simulink library "utility_service_lib"  (Simulink 8.1)
settings: Solver=ode45  StartTime=0.0  StopTime=10.0  RelTol=1e-3
values from neighbouring files (symbols this model uses):
  Ts = 100E-6    (= 0.0001)    [BANSHEE_init.m]
undefined symbols (not defined in the file or in its folder): Left, type, V
libraries: simulink x10, rtlab x10, RMS_lib x10, cables_lib x8, breaker_lib x4, transformer_lib x3, EasyGen3500_GensetSignalScaling_lib x2, PQFV_lib x2, Banshee_SEL751_Woodward_lib x1, SEL751_SignalScaling_lib x1, ssn_lib x1, TestSeq_slave_lib x1
settings Model: Creator=RE25624  LastModifiedBy=re25624

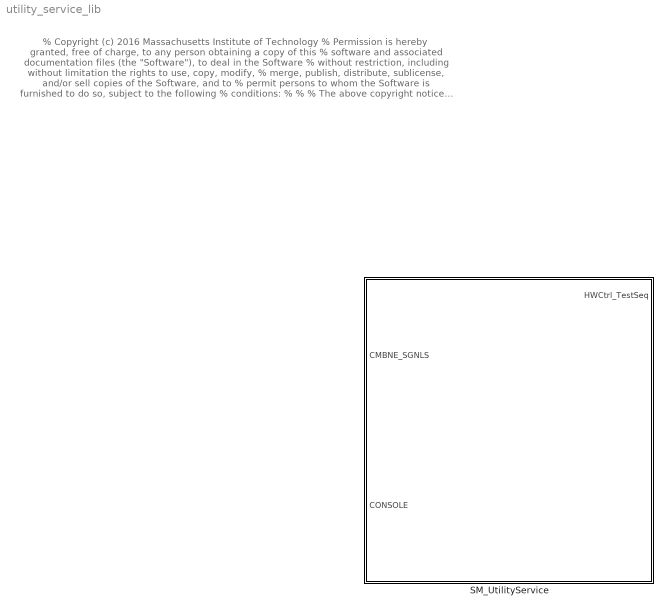
== system utility_service_lib ==
  note: % Copyright (c) 2016 Massachusetts Institute of Technology
      | % Permission is hereby granted, free of charge, to any person obtaining a copy of this
      | % software and associated documentation files (the "Software"), to deal in the Software
      | % without restriction, including without limitation the rights to use, copy, modify,
      | % merge, publish, distribute, sublicense, and/or sell copies of the Software, and to
      | % permit persons to whom the Software is furnished to do so, subject to the following
      | % conditions:
      | %
      | %
      | % The above copyright notice and this permission notice shall be included in
      | % all copies or substantial portions of the Software.
      | %
      | % THE SOFTWARE IS PROVIDED "AS IS", WITHOUT WARRANTY OF ANY KIND, EXPRESS OR IMPLIED,
      | % INCLUDING BUT NOT LIMITED TO THE WARRANTIES OF MERCHANTABILITY, FITNESS FOR A
      | % PARTICULAR PURPOSE AND NONINFRINGEMENT. IN NO EVENT SHALL THE AUTHORS OR COPYRIGHT
      | % HOLDERS BE LIABLE FOR ANY CLAIM, DAMAGES OR OTHER LIABILITY, WHETHER IN AN ACTION
      | % OF CONTRACT, TORT OR OTHERWISE, ARISING FROM, OUT OF OR IN CONNECTION WITH THE
      | % SOFTWARE OR THE USE OR OTHER DEALINGS IN THE SOFTWARE.
      | %
      | %
      | %%
  SM_UtilityService : Subsystem

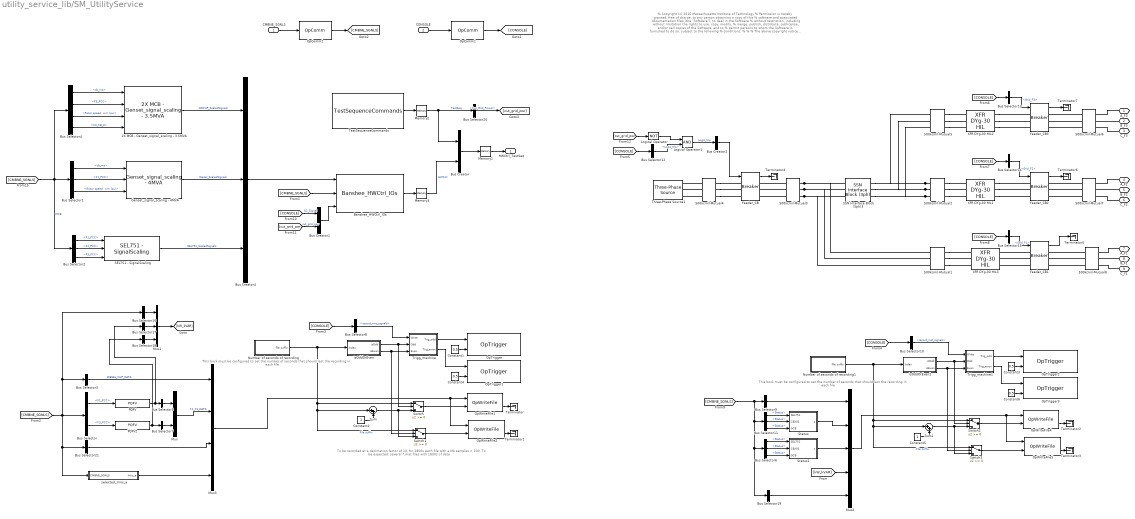
== system utility_service_lib/SM_UtilityService ==
  note: This bock must be configured to set the number of
      | seconds that should last the recording in each file
  note: To be recorded at a decimation factor of 10,   for 1800s each file with a Nb samples = 200.
      | To be expected: several *.mat files with 1800s of data
  note: This bock must be configured to set the number of
      | seconds that should last the recording in each file
  note: % Copyright (c) 2016 Massachusetts Institute of Technology
      | % Permission is hereby granted, free of charge, to any person obtaining a copy of this
      | % software and associated documentation files (the "Software"), to deal in the Software
      | % without restriction, including without limitation the rights to use, copy, modify,
      | % merge, publish, distribute, sublicense, and/or sell copies of the Software, and to
      | % permit persons to whom the Software is furnished to do so, subject to the following
      | % conditions:
      | %
      | %
      | % The above copyright notice and this permission notice shall be included in
      | % all copies or substantial portions of the Software.
      | %
      | % THE SOFTWARE IS PROVIDED "AS IS", WITHOUT WARRANTY OF ANY KIND, EXPRESS OR IMPLIED,
      | % INCLUDING BUT NOT LIMITED TO THE WARRANTIES OF MERCHANTABILITY, FITNESS FOR A
      | % PARTICULAR PURPOSE AND NONINFRINGEMENT. IN NO EVENT SHALL THE AUTHORS OR COPYRIGHT
      | % HOLDERS BE LIABLE FOR ANY CLAIM, DAMAGES OR OTHER LIABILITY, WHETHER IN AN ACTION
      | % OF CONTRACT, TORT OR OTHERWISE, ARISING FROM, OUT OF OR IN CONNECTION WITH THE
      | % SOFTWARE OR THE USE OR OTHER DEALINGS IN THE SOFTWARE.
      | %
      | %
      | %%
  CMBNE_SGNLS : Inport
  CONSOLE : Inport  Port=2
  2X MCB - Genset_signal_scaling - 3.5MVA : EasyGen3500_GensetSignalScaling_lib/2X MCB - Genset_signal_scaling - 3.5MVA  Vpk_mcb=11268  watt_mcb=3150000  Vpk_gcb=11268  watt_gcb=3150000  rated_rpm=1800  wm_noise_bias=0.02
  500kcmil-Mutual1 : cables_lib/500kcmil-Mutual  length=200  par_sets=1  ratio=3
  500kcmil-Mutual2 : cables_lib/500kcmil-Mutual  length=200  par_sets=1  ratio=3
  500kcmil-Mutual{3..4,6..8} (5 alike) : cables_lib/500kcmil-Mutual  length=50  par_sets=1  ratio=3
  500kcmil-Mutual5 : cables_lib/500kcmil-Mutual  length=200  par_sets=1  ratio=3
  Banshee_HWCtrl_IOs : Banshee_SEL751_Woodward_lib/Banshee_HWCtrl_IOs  SystemSampleTime=-1
  Bus Creator : BusCreator  Inputs=2
  Bus Creator1 : BusCreator  Inputs=2
  Bus Creator2 : BusCreator  Inputs=1
  Bus Creator4 : BusCreator  Inputs=3
  Bus Selector : BusSelector  OutputSignals=F1_MS_IN.CB_DATA.F1_PCC,F3_MS_IN.CB_DATA.F3_PCC
  Bus Selector1 : BusSelector  OutputSignals="F1_MS_IN.DIESEL_DATA.DIESEL_GCB.cb_ms,F1_MS_IN.CB_DATA.F1_PCC,F1_MS_IN.DIESEL_DATA.Gen2_meas.w.w.Rotor speed  wm (pu)"
  Bus Selector10 : BusSelector  OutputSignals=DataLogging.record_inst_signals
  Bus Selector11 : BusSelector  OutputSignals=F1_MS_IN.CB_DATA.F1_PCC.Status,F1_MS_IN.CB_DATA.F1_CB_3.Status,F1_MS_IN.DIESEL_DATA.DIESEL_GCB.cb_ms.Status
  Bus Selector12 : BusSelector  OutputSignals=GridStatusCtrl.Substation.Logic_trip
  Bus Selector13 : BusSelector  OutputSignals=GridStatusCtrl.Grid_F3
  Bus Selector14 : BusSelector  OutputSignals=GridStatusCtrl.Grid_F2
  Bus Selector15 : BusSelector  OutputSignals=GridStatusCtrl.Grid_F1
  Bus Selector16 : BusSelector  OutputSignals=F1_MS_IN.DIESEL_DATA.DIESEL_GCB.kw,F1_MS_IN.DIESEL_DATA.DIESEL_GCB.kvar,F3_MS_IN.NG_CHP_DATA.NG_CHP_GCB.kw,F3_MS_IN.NG_CHP_DATA.NG_CHP_GCB.kvar  OutputAsBus=on
  Bus Selector17 : BusSelector  OutputSignals=kw,kvar  OutputAsBus=on
  Bus Selector18 : BusSelector  OutputSignals=kw,kvar  OutputAsBus=on
  Bus Selector19 : BusSelector  OutputSignals=F1_MS_IN.DIESEL_DATA.DIESEL_GCB.cb_ms.Iabc,F3_MS_IN.NG_CHP_DATA.NG_CHP_GCB.cb_ms.Iabc,F1_MS_IN.DIESEL_DATA.Gen2_meas.Vf.vf,F3_MS_IN.NG_CHP_DATA.Gen1_meas.Vf.vf  OutputAsBus=on
  Bus Selector2 : BusSelector  OutputSignals=F1_MS_IN.CB_DATA.F1_PCC,F2_MS_IN.CB_DATA.F2_PCC,F3_MS_IN.CB_DATA.F3_PCC
  Bus Selector20 : BusSelector  OutputSignals=Cut_Grid_Power
  Bus Selector21 : BusSelector  OutputSignals=F1_RELAY_OUT.F1_CB_1.m.status,F1_RELAY_OUT.F1_CB_2.m.status,F1_RELAY_OUT.F1_CB_3.m.status,F1_RELAY_OUT.F1_CB_4.m.status,F1_RELAY_OUT.F1_CB_5.m.status,F1_RELAY_OUT.F1_CB_6.m.status,F1_RELAY_OUT.F1_CB_7.m.status,F1_RELAY_OUT.F1_CB_8.m.status,F1_RELAY_OUT.F1_CB_9.m.status,F1_RELAY_OUT.F1_CB_10.m.status,F1_RELAY_OUT.F1_CB_11.m.status,F1_RELAY_OUT.F1_CB_12.m.status,F1_RELAY_OUT.F1_CB_13.m.status,F1_RELAY_OUT.F1_CB_14.m.status,F2_RELAY_OUT.F2_CB_1.m.status,F2_RELAY_OUT.F2_CB_2.m.status,F2_RELAY_OUT.F2_CB_3.m.status,F2_RELAY_OUT.F2_CB_4.m.status,F2_RELAY_OUT.F2_CB_5.m.status,F2_RELAY_OUT.F2_CB_6.m.status,F2_RELAY_OUT.F2_CB_7.m.status,F2_RELAY_OUT.F2_CB_8.m.status,F2_RELAY_OUT.F2_CB_9.m.status,F2_RELAY_OUT.F2_CB_10.m.status,F2_RELAY_OUT.F2_CB_11.m.status,F2_RELAY_OUT.F2_CB_12.m.status,F2_RELAY_OUT.F2_CB_13.m.status,F2_RELAY_OUT.F2_CB_14.m.status,F2_RELAY_OUT.F2_CB_15.m.status,F2_RELAY_OUT.F2_CB_16.m.status,F2_RELAY_OUT.F2_CB_17.m.status,F2_RELAY_OUT.F2_CB_18.m.status,F2_RELAY_OUT.F2_CB_19.m.status,F3_RELAY_OUT.F3_CB_1.m.status,F3_RELAY_OUT.F3_CB_2.m.status,F3_RELAY_OUT.F3_CB_3.m.status,F3_RELAY_OUT.F3_CB_4.m.status,F3_RELAY_OUT.F3_CB_5.m.status,F3_RELAY_OUT.F3_CB_6.m.status,F3_RELAY_OUT.F3_CB_7.m.status,F3_RELAY_OUT.F3_CB_8.m.status,F3_RELAY_OUT.F3_CB_9.m.status  OutputAsBus=on
  Bus Selector3 : BusSelector  OutputSignals=F1_MS_IN.DIESEL_DATA.DIESEL_GCB.VRMSLL,F1_MS_IN.DIESEL_DATA.DIESEL_GCB.Freq,F1_MS_IN.DIESEL_DATA.DIESEL_GCB.kw,F1_MS_IN.DIESEL_DATA.DIESEL_GCB.kvar,F3_MS_IN.NG_CHP_DATA.NG_CHP_GCB.VRMSLL,F3_MS_IN.NG_CHP_DATA.NG_CHP_GCB.Freq,F3_MS_IN.NG_CHP_DATA.NG_CHP_GCB.kw,F3_MS_IN.NG_CHP_DATA.NG_CHP_GCB.kvar  OutputAsBus=on
  Bus Selector4 : BusSelector  OutputSignals="F3_MS_IN.NG_CHP_DATA.NG_CHP_GCB.cb_ms,F3_MS_IN.CB_DATA.F3_PCC,F3_MS_IN.NG_CHP_DATA.Gen1_meas.w.w.Rotor speed  wm (pu),F3_MS_IN.CB_DATA.F3_CB_3"
  Bus Selector5 : BusSelector  OutputSignals=VRMSLL,Freq,kw,kvar  OutputAsBus=on
  Bus Selector6 : BusSelector  OutputSignals=F3_MS_IN.CB_DATA.F3_PCC.Status,F3_MS_IN.CB_DATA.F3_CB_3.Status,F3_MS_IN.NG_CHP_DATA.NG_CHP_GCB.cb_ms.Status
  Bus Selector7 : BusSelector  OutputSignals=VRMSLL,Freq,kw,kvar  OutputAsBus=on
  Bus Selector8 : BusSelector  OutputSignals=DataLogging.record_rms_signals
  Bus Selector9 : BusSelector  OutputSignals=F1_MS_IN.CB_DATA.F1_PCC.Vabc_bus,F3_MS_IN.CB_DATA.F3_PCC.Vabc_bus,F1_MS_IN.DIESEL_DATA.DIESEL_GCB.cb_ms.Vabc_bus,F3_MS_IN.NG_CHP_DATA.NG_CHP_GCB.cb_ms.Vabc_bus  OutputAsBus=on
  Constant{1,3..4,6} (4 alike) : Constant  Value=0.5
  Constant2 : Constant
  Constant5 : Constant
  Feeder_CB{,1..3} (4 alike) : breaker_lib/Breaker  Ts=Ts  mech_delay=cb_mech_delay
  Genset_signal_scaling - 4MVA : EasyGen3500_GensetSignalScaling_lib/Genset_signal_scaling - 4MVA  Vpk_mcb=11268  watt_mcb=3600000  Vpk_gcb=11268  watt_gcb=3600000  rated_rpm=1800  wm_noise_bias=0.02
  Logical Operator : Logic  Operator=NOT  AllPortsSameDT=off  OutDataTypeStr=boolean
  Logical Operator1 : Logic  AllPortsSameDT=off  OutDataTypeStr=boolean
  Memory1 : Memory
  Memory2 : Memory
  Memory3 : Memory
  Mux : Mux  Inputs=2
  Mux1 : Mux  Inputs=3
  Mux2 : Mux  Inputs=5
  Mux3 : Mux
  Number of seconds of recording : Subsystem  mask{time_s=1800}
      mask prompts: time_s "Time in seconds"
      mask help: Set the number of seconds that should last the recording in each file.
  Number of seconds of recording1 : Subsystem  mask{time_s=300}
      mask prompts: time_s "Time in seconds"
      mask help: Set the number of seconds that should last the recording in each file.
  OpComm1 : rtlab/OpComm  nbport=1  groupe_acq=1  subsys_rate=0  st=0  Synchronization=on  Interpolation=on  Threshold=1.0  Missed_Data=off  Sim_Time=off  Samples=off  dynSigOut=off  from_console=1  warning_done=off  writeOpCommFile=off  Offset=off
  OpComm2 : rtlab/OpComm  nbport=1  groupe_acq=1  subsys_rate=0  st=0  Synchronization=on  Interpolation=on  Threshold=1.0  Missed_Data=off  Sim_Time=off  Samples=off  dynSigOut=off  from_console=0  warning_done=off  writeOpCommFile=off  Offset=off
  OpTrigger : rtlab/DataLogging/OpTrigger  Trig_Type=TRIGGER SIGNAL >= TRIGGER LEVEL  Trig_Offset=0  Acq_Group=28
  OpTrigger1 : rtlab/DataLogging/OpTrigger  Trig_Type=TRIGGER SIGNAL >= TRIGGER LEVEL  Trig_Offset=0  Acq_Group=29
  OpTrigger2 : rtlab/DataLogging/OpTrigger  Trig_Type=TRIGGER SIGNAL >= TRIGGER LEVEL  Trig_Offset=0  Acq_Group=26
  OpTrigger3 : rtlab/DataLogging/OpTrigger  Trig_Type=TRIGGER SIGNAL >= TRIGGER LEVEL  Trig_Offset=0  Acq_Group=27
  OpWriteFile1 : rtlab/DataLogging/OpWriteFile  Static_File=off  varname=recVar  Filename=A_FILE_RECORDED_o.mat  rtpath='./'  nrtpath='.\'  Acq_Group=28  file_size=150000000  write_offline=off  Sim_Mode=off  Nb_Samples=1000  Buffer_size=0
      settings: Decimation=20
  OpWriteFile2 : rtlab/DataLogging/OpWriteFile  Static_File=off  varname=recVar  Filename=A_FILE_RECORDED_e.mat  rtpath='./'  nrtpath='.\'  Acq_Group=29  file_size=150000000  write_offline=off  Sim_Mode=off  Nb_Samples=1000  Buffer_size=0
      settings: Decimation=20
  OpWriteFile4 : rtlab/DataLogging/OpWriteFile  Static_File=off  varname=recVar  Filename=A_INST_RECORDED_o.mat  rtpath='./'  nrtpath='.\'  Acq_Group=26  file_size=150000000  write_offline=off  Sim_Mode=off  Nb_Samples=1000  Buffer_size=0
      settings: Decimation=4
  OpWriteFile5 : rtlab/DataLogging/OpWriteFile  Static_File=off  varname=recVar  Filename=A_INST_RECORDED_e.mat  rtpath='./'  nrtpath='.\'  Acq_Group=27  file_size=150000000  write_offline=off  Sim_Mode=off  Nb_Samples=1000  Buffer_size=0
      settings: Decimation=4
  PQFV : PQFV_lib/PQFV  VRMSLL=13800
  PQFV2 : PQFV_lib/PQFV  VRMSLL=13800
  SEL751 - SignalScaling : SEL751_SignalScaling_lib/SEL751 - SignalScaling  ct_ratio=1/1250  pt_ratio=1/1800
  SSN Interface Block (3ph)3 : ssn_lib/SSN Interface Block (3ph)  nb_phase=3  nb_port=2  p1_type=V-type(Left)  p2_type=V-type (Right)  p3_type=V-type(Left)  p4_type=V-type(Left)  p5_type=V-type(Left)  p6_type=V-type(Left)  p7_type=V-type(Left)  p8_type=V-type(Left)  p9_type=V-type(Left)  p10_type=V-type(Left)  p11_type=V-type(Left)  p12_type=V-type(Left)  p13_type=V-type(Left)  p14_type=V-type(Left)  p15_type=V-type(Left)  p16_type=V-type(Left)  I_port_shunt_resistance=1e9
  Status : Subsystem
  Status1 : Subsystem
  Sum : Sum  Inputs=|++
  Sum1 : Sum  Inputs=|++
  Switch{,1..3} (4 alike) : Switch
  Terminator{,1..7} (8 alike) : Terminator
  TestSequenceCommands : TestSeq_slave_lib/TestSequenceCommands
  Three-Phase Source1 : powerlib/Electrical Sources/Three-Phase Source  Voltage=115000  PhaseAngle=0  Frequency=60  InternalConnection=Yg  SpecifyImpedance=on  Resistance=0.8929  Inductance=16.58e-3  ShortCircuitLevel=2000e6  BaseVoltage=115000  XRratio=100  BusType=swing  Pref=0  Qref=0  Qmin=-inf  Qmax=inf
  Trigg_machine : Subsystem
  Trigg_machine1 : Subsystem
  XFR DYg-30 HIL1 : transformer_lib/XFR DYg-30 HIL  Rating=50000  Vp=115000  Vs=13800  Z=6  XR=30
  XFR DYg-30 HIL2 : transformer_lib/XFR DYg-30 HIL  Rating=50000  Vp=115000  Vs=13800  Z=6  XR=30
  XFR DYg-30 HIL3 : transformer_lib/XFR DYg-30 HIL  Rating=50000  Vp=115000  Vs=13800  Z=6  XR=30
  isOddOrEven : Subsystem
  isOddOrEven1 : Subsystem
  selected_Irms_a : Subsystem
  A_F3 : PMIOPort  Port=1  Side=Right
  B_F3 : PMIOPort  Port=2  Side=Right
  C_F3 : PMIOPort  Port=3  Side=Right
  A_F2 : PMIOPort  Port=4  Side=Right
  B_F2 : PMIOPort  Port=5  Side=Right
  C_F2 : PMIOPort  Port=6  Side=Right
  A_F1 : PMIOPort  Port=7  Side=Right
  B_F1 : PMIOPort  Port=8  Side=Right
  C_F1 : PMIOPort  Port=9  Side=Right
  HWCtrl_TestSeq : Outport
  wires:
  Bus Creator2/1 -> Feeder_CB/1
  Logical Operator1/1 -> Bus Creator2/1  "Logic_trip"
  Logical Operator/1 -> Logical Operator1/1
  [cut_grid_pwr] -> Logical Operator/1
  [cut_grid_pwr] -> Bus Creator1/2  "cut_grid_pwr"
  Bus Selector20/1 -> [cut_grid_pwr]  "<Cut_Grid_Power>"
  Bus Creator1/1 -> Banshee_HWCtrl_IOs/3
  selected_Irms_a/1(Irms_a) -> Mux3/4
  Bus Creator/1 -> Memory1/1
  Memory2/1 -> Bus Selector20/1, Bus Creator/1  "TestSeq"
  Memory3/1 -> Bus Creator/2  "HWCtrl"
  TestSequenceCommands/1 -> Memory2/1
  Banshee_HWCtrl_IOs/1 -> Memory3/1
  Memory1/1 -> HWCtrl_TestSeq/1
  Bus Selector21/1 -> Mux3/3
  Bus Selector19/1 -> Mux2/5
  [kW_kVAR] -> Mux2/4
  Mux1/1 -> [kW_kVAR]
  Bus Selector18/1 -> Mux1/3
  Bus Selector17/1 -> Mux1/2
  Bus Selector16/1 -> Mux1/1
  PQFV2/1 -> Bus Selector7/1, Bus Selector18/1
  PQFV/1 -> Bus Selector5/1, Bus Selector17/1
  Status1/1(o) -> Mux2/3
  Status/1(o) -> Mux2/2
  Bus Selector6/3 -> Status1/3(GCB)  "<Status>"
  Bus Selector6/2 -> Status1/2(CBX03)  "<Status>"
  Bus Selector6/1 -> Status1/1(SEL751)  "<Status>"
  Bus Selector11/3 -> Status/3(GCB)  "<Status>"
  Bus Selector11/2 -> Status/2(CBX03)  "<Status>"
  Bus Selector11/1 -> Status/1(SEL751)  "<Status>"
  [CONSOLE] -> Bus Creator1/1  "SC_Signal"
  Bus Selector9/1 -> Mux2/1
  [CMBNE_SGNLS] -> Bus Selector9/1, Bus Selector11/1, Bus Selector6/1, Bus Selector19/1
  Bus Selector15/1 -> Feeder_CB1/1  "<Grid_F1>"
  Bus Selector14/1 -> Feeder_CB2/1  "<Grid_F2>"
  Bus Selector13/1 -> Feeder_CB3/1  "<Grid_F3>"
  Bus Selector12/1 -> Logical Operator1/2  "<Logic_trip>"
  Feeder_CB3/1 -> Terminator7/1
  Feeder_CB2/1 -> Terminator6/1
  Feeder_CB1/1 -> Terminator5/1
  [CONSOLE] -> Bus Selector15/1
  [CONSOLE] -> Bus Selector14/1
  [CONSOLE] -> Bus Selector13/1
  [CONSOLE] -> Bus Selector12/1
  Feeder_CB/1 -> Terminator4/1
  [CMBNE_SGNLS] -> Bus Selector/1, Bus Selector21/1, selected_Irms_a/1(CMBNE_SGNLS), Bus Selector3/1, Bus Selector16/1
  [CONSOLE] -> Bus Selector10/1
  OpWriteFile5/2 -> Terminator3/1
  OpWriteFile4/2 -> Terminator2/1
  Bus Selector10/1 -> Trigg_machine1/1(Write)  "<record_inst_signals>"
  Number of seconds of recording1/1(file suffix) -> isOddOrEven1/1(Index), Sum1/1, Switch3/1, Switch2/1  "File suffix"
  Sum1/1 -> Switch2/3, Switch3/3
  Constant5/1 -> Sum1/2
  Switch3/1 -> OpWriteFile5/2
  Switch2/1 -> OpWriteFile4/2
  isOddOrEven1/2(isEven) -> Switch3/2, Trigg_machine1/3(Even)
  isOddOrEven1/1(isOdd) -> Switch2/2, Trigg_machine1/2(Odd)
  Constant6/1 -> OpTrigger3/2
  Constant3/1 -> OpTrigger2/2
  Trigg_machine1/2(Trig_even) -> OpTrigger3/1
  Trigg_machine1/1(Trig_odd) -> OpTrigger2/1
  Mux2/1 -> OpWriteFile4/1, OpWriteFile5/1
  [CONSOLE] -> Bus Selector8/1
  OpComm1/1 -> [CONSOLE]
  CONSOLE/1 -> OpComm1/1
  Mux/1 -> Mux3/2  "F1_F3_DATA"
  Bus Selector3/1 -> Mux3/1  "DIESEL_CHP_DATA"
  Bus Selector5/1 -> Mux/1
  Bus Selector7/1 -> Mux/2
  Bus Selector/2 -> PQFV2/1  "<F3_PCC>"
  Bus Selector/1 -> PQFV/1  "<F1_PCC>"
  OpWriteFile2/2 -> Terminator1/1
  OpWriteFile1/2 -> Terminator/1
  Bus Selector8/1 -> Trigg_machine/1(Write)  "<record_rms_signals>"
  Number of seconds of recording/1(file suffix) -> isOddOrEven/1(Index), Sum/1, Switch1/1, Switch/1  "File suffix"
  Sum/1 -> Switch/3, Switch1/3
  Constant2/1 -> Sum/2
  Switch1/1 -> OpWriteFile2/2
  Switch/1 -> OpWriteFile1/2
  isOddOrEven/2(isEven) -> Switch1/2, Trigg_machine/3(Even)
  isOddOrEven/1(isOdd) -> Switch/2, Trigg_machine/2(Odd)
  Constant4/1 -> OpTrigger1/2
  Constant1/1 -> OpTrigger/2
  Trigg_machine/2(Trig_even) -> OpTrigger1/1
  Trigg_machine/1(Trig_odd) -> OpTrigger/1
  Mux3/1 -> OpWriteFile1/1, OpWriteFile2/1
  [CMBNE_SGNLS] -> Banshee_HWCtrl_IOs/2
  Bus Selector4/4 -> 2X MCB - Genset_signal_scaling - 3.5MVA/4  "<F3_CB_3>"
  Bus Selector2/3 -> SEL751 - SignalScaling/3  "<F3_PCC>"
  Bus Selector2/1 -> SEL751 - SignalScaling/1  "<F1_PCC>"
  Bus Selector2/2 -> SEL751 - SignalScaling/2  "<F2_PCC>"
  SEL751 - SignalScaling/1 -> Bus Creator4/3  "SEL751_ScaledSignals"
  OpComm2/1 -> [CMBNE_SGNLS]
  CMBNE_SGNLS/1 -> OpComm2/1
  Bus Selector1/1 -> Genset_signal_scaling - 4MVA/1  "<cb_ms>"
  Bus Selector1/2 -> Genset_signal_scaling - 4MVA/2  "<F1_PCC>"
  Bus Selector1/3 -> Genset_signal_scaling - 4MVA/3  "<Rotor speed  wm (pu)>"
  Bus Creator4/1 -> Banshee_HWCtrl_IOs/1
  Bus Selector4/1 -> 2X MCB - Genset_signal_scaling - 3.5MVA/1  "<cb_ms>"
  Bus Selector4/2 -> 2X MCB - Genset_signal_scaling - 3.5MVA/2  "<F3_PCC>"
  Bus Selector4/3 -> 2X MCB - Genset_signal_scaling - 3.5MVA/3  "<Rotor speed  wm (pu)>"
  [CMBNE_SGNLS] -> Bus Selector1/1, Bus Selector2/1, Bus Selector4/1  "MCB"
  Genset_signal_scaling - 4MVA/1 -> Bus Creator4/2  "Diesel_ScaledSignals"
  2X MCB - Genset_signal_scaling - 3.5MVA/1 -> Bus Creator4/1  "NGCHP_ScaledSignals"
  connections:
  C_F3/RConn1 -- 500kcmil-Mutual6/RConn3
  A_F3/RConn1 -- 500kcmil-Mutual6/RConn1
  B_F3/RConn1 -- 500kcmil-Mutual6/RConn2
  C_F2/RConn1 -- 500kcmil-Mutual7/RConn3
  A_F2/RConn1 -- 500kcmil-Mutual7/RConn1
  B_F2/RConn1 -- 500kcmil-Mutual7/RConn2
  A_F1/RConn1 -- 500kcmil-Mutual8/RConn1
  C_F1/RConn1 -- 500kcmil-Mutual8/RConn3
  B_F1/RConn1 -- 500kcmil-Mutual8/RConn2
  500kcmil-Mutual8/LConn3 -- Feeder_CB1/RConn3
  500kcmil-Mutual8/LConn2 -- Feeder_CB1/RConn2
  500kcmil-Mutual8/LConn1 -- Feeder_CB1/RConn1
  500kcmil-Mutual7/LConn1 -- Feeder_CB2/RConn1
  500kcmil-Mutual7/LConn3 -- Feeder_CB2/RConn3
  500kcmil-Mutual7/LConn2 -- Feeder_CB2/RConn2
  500kcmil-Mutual6/LConn1 -- Feeder_CB3/RConn1
  500kcmil-Mutual6/LConn3 -- Feeder_CB3/RConn3
  500kcmil-Mutual6/LConn2 -- Feeder_CB3/RConn2
  Feeder_CB1/LConn1 -- XFR DYg-30 HIL3/RConn1
  Feeder_CB1/LConn2 -- XFR DYg-30 HIL3/RConn2
  Feeder_CB1/LConn3 -- XFR DYg-30 HIL3/RConn3
  XFR DYg-30 HIL1/RConn1 -- Feeder_CB2/LConn1
  XFR DYg-30 HIL1/RConn2 -- Feeder_CB2/LConn2
  XFR DYg-30 HIL1/RConn3 -- Feeder_CB2/LConn3
  XFR DYg-30 HIL2/RConn3 -- Feeder_CB3/LConn3
  XFR DYg-30 HIL2/RConn2 -- Feeder_CB3/LConn2
  XFR DYg-30 HIL2/RConn1 -- Feeder_CB3/LConn1
  500kcmil-Mutual2/LConn3 -- 500kcmil-Mutual5/LConn3 -- SSN Interface Block (3ph)3/RConn3
  500kcmil-Mutual2/LConn2 -- 500kcmil-Mutual5/LConn2 -- SSN Interface Block (3ph)3/RConn2
  500kcmil-Mutual2/LConn1 -- 500kcmil-Mutual5/LConn1 -- SSN Interface Block (3ph)3/RConn1
  500kcmil-Mutual1/RConn1 -- XFR DYg-30 HIL3/LConn1
  500kcmil-Mutual1/RConn2 -- XFR DYg-30 HIL3/LConn2
  500kcmil-Mutual1/RConn3 -- XFR DYg-30 HIL3/LConn3
  500kcmil-Mutual5/RConn3 -- XFR DYg-30 HIL2/LConn3
  500kcmil-Mutual5/RConn1 -- XFR DYg-30 HIL2/LConn1
  500kcmil-Mutual5/RConn2 -- XFR DYg-30 HIL2/LConn2
  500kcmil-Mutual2/RConn3 -- XFR DYg-30 HIL1/LConn3
  500kcmil-Mutual2/RConn1 -- XFR DYg-30 HIL1/LConn1
  500kcmil-Mutual2/RConn2 -- XFR DYg-30 HIL1/LConn2
  500kcmil-Mutual4/LConn2 -- Three-Phase Source1/RConn2
  500kcmil-Mutual4/LConn1 -- Three-Phase Source1/RConn1
  500kcmil-Mutual4/LConn3 -- Three-Phase Source1/RConn3
  500kcmil-Mutual4/RConn1 -- Feeder_CB/LConn1
  500kcmil-Mutual4/RConn2 -- Feeder_CB/LConn2
  500kcmil-Mutual4/RConn3 -- Feeder_CB/LConn3
  500kcmil-Mutual3/RConn3 -- 500kcmil-Mutual1/LConn3 -- SSN Interface Block (3ph)3/LConn3
  500kcmil-Mutual3/RConn1 -- 500kcmil-Mutual1/LConn1 -- SSN Interface Block (3ph)3/LConn1
  500kcmil-Mutual3/RConn2 -- 500kcmil-Mutual1/LConn2 -- SSN Interface Block (3ph)3/LConn2
  500kcmil-Mutual3/LConn2 -- Feeder_CB/RConn2
  500kcmil-Mutual3/LConn1 -- Feeder_CB/RConn1
  500kcmil-Mutual3/LConn3 -- Feeder_CB/RConn3

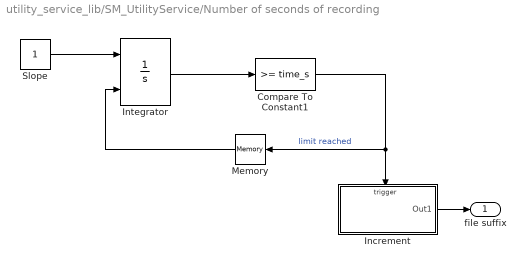
== system utility_service_lib/SM_UtilityService/Number of seconds of recording ==
  Compare To Constant1 : simulink/Logic and Bit Operations/Compare To Constant  relop=>=  const=time_s  OutDataTypeStr=boolean
  Increment : Subsystem
  Integrator : Integrator  ExternalReset=rising
  Memory : Memory
  Slope : Constant
  file suffix : Outport
  wires:
  Slope/1 -> Integrator/1
  Integrator/1 -> Compare To Constant1/1
  Compare To Constant1/1 -> Memory/1, Increment/Trigger  "limit reached"
  Memory/1 -> Integrator/2
  Increment/1(Out1) -> file suffix/1

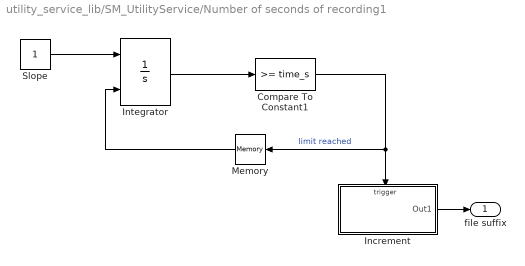
== system utility_service_lib/SM_UtilityService/Number of seconds of recording1 ==
  Compare To Constant1 : simulink/Logic and Bit Operations/Compare To Constant  relop=>=  const=time_s  OutDataTypeStr=boolean
  Increment : Subsystem
  Integrator : Integrator  ExternalReset=rising
  Memory : Memory
  Slope : Constant
  file suffix : Outport
  wires:
  Slope/1 -> Integrator/1
  Integrator/1 -> Compare To Constant1/1
  Compare To Constant1/1 -> Memory/1, Increment/Trigger  "limit reached"
  Memory/1 -> Integrator/2
  Increment/1(Out1) -> file suffix/1

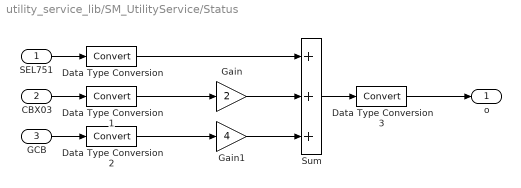
== system utility_service_lib/SM_UtilityService/Status ==
  SEL751 : Inport
  CBX03 : Inport  Port=2
  GCB : Inport  Port=3
  Data Type Conversion{,1..3} (4 alike) : DataTypeConversion
  Gain : Gain  Gain=2
  Gain1 : Gain  Gain=4
  Sum : Sum  Inputs=+++
  o : Outport
  wires:
  Data Type Conversion3/1 -> o/1
  Data Type Conversion2/1 -> Gain1/1
  Data Type Conversion1/1 -> Gain/1
  Data Type Conversion/1 -> Sum/1
  Sum/1 -> Data Type Conversion3/1
  Gain1/1 -> Sum/3
  Gain/1 -> Sum/2
  SEL751/1 -> Data Type Conversion/1
  CBX03/1 -> Data Type Conversion1/1
  GCB/1 -> Data Type Conversion2/1

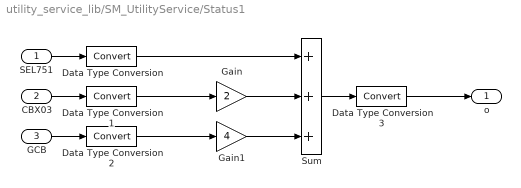
== system utility_service_lib/SM_UtilityService/Status1 ==
  SEL751 : Inport
  CBX03 : Inport  Port=2
  GCB : Inport  Port=3
  Data Type Conversion{,1..3} (4 alike) : DataTypeConversion
  Gain : Gain  Gain=2
  Gain1 : Gain  Gain=4
  Sum : Sum  Inputs=+++
  o : Outport
  wires:
  Data Type Conversion3/1 -> o/1
  Data Type Conversion2/1 -> Gain1/1
  Data Type Conversion1/1 -> Gain/1
  Data Type Conversion/1 -> Sum/1
  Sum/1 -> Data Type Conversion3/1
  Gain1/1 -> Sum/3
  Gain/1 -> Sum/2
  SEL751/1 -> Data Type Conversion/1
  CBX03/1 -> Data Type Conversion1/1
  GCB/1 -> Data Type Conversion2/1

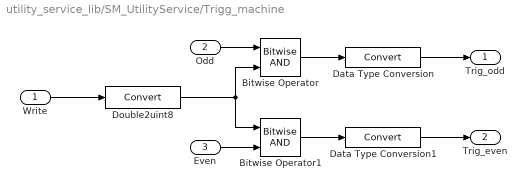
== system utility_service_lib/SM_UtilityService/Trigg_machine ==
  Write : Inport
  Odd : Inport  Port=2
  Even : Inport  Port=3
  Bitwise Operator : simulink/Logic and Bit Operations/Bitwise Operator  logicop=AND  UseBitMask=off  NumInputPorts=2  BitMask=bin2dec('11011001')  BitMaskRealWorld=Stored Integer
  Bitwise Operator1 : simulink/Logic and Bit Operations/Bitwise Operator  logicop=AND  UseBitMask=off  NumInputPorts=2  BitMask=bin2dec('11011001')  BitMaskRealWorld=Stored Integer
  Data Type Conversion : DataTypeConversion
  Data Type Conversion1 : DataTypeConversion
  Double2uint8 : DataTypeConversion
  Trig_odd : Outport
  Trig_even : Outport  Port=2
  wires:
  Double2uint8/1 -> Bitwise Operator1/1, Bitwise Operator/2
  Write/1 -> Double2uint8/1
  Odd/1 -> Bitwise Operator/1
  Data Type Conversion1/1 -> Trig_even/1
  Data Type Conversion/1 -> Trig_odd/1
  Even/1 -> Bitwise Operator1/2
  Bitwise Operator1/1 -> Data Type Conversion1/1
  Bitwise Operator/1 -> Data Type Conversion/1

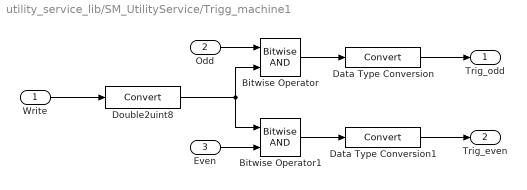
== system utility_service_lib/SM_UtilityService/Trigg_machine1 ==
  Write : Inport
  Odd : Inport  Port=2
  Even : Inport  Port=3
  Bitwise Operator : simulink/Logic and Bit Operations/Bitwise Operator  logicop=AND  UseBitMask=off  NumInputPorts=2  BitMask=bin2dec('11011001')  BitMaskRealWorld=Stored Integer
  Bitwise Operator1 : simulink/Logic and Bit Operations/Bitwise Operator  logicop=AND  UseBitMask=off  NumInputPorts=2  BitMask=bin2dec('11011001')  BitMaskRealWorld=Stored Integer
  Data Type Conversion : DataTypeConversion
  Data Type Conversion1 : DataTypeConversion
  Double2uint8 : DataTypeConversion
  Trig_odd : Outport
  Trig_even : Outport  Port=2
  wires:
  Double2uint8/1 -> Bitwise Operator1/1, Bitwise Operator/2
  Write/1 -> Double2uint8/1
  Odd/1 -> Bitwise Operator/1
  Data Type Conversion1/1 -> Trig_even/1
  Data Type Conversion/1 -> Trig_odd/1
  Even/1 -> Bitwise Operator1/2
  Bitwise Operator1/1 -> Data Type Conversion1/1
  Bitwise Operator/1 -> Data Type Conversion/1

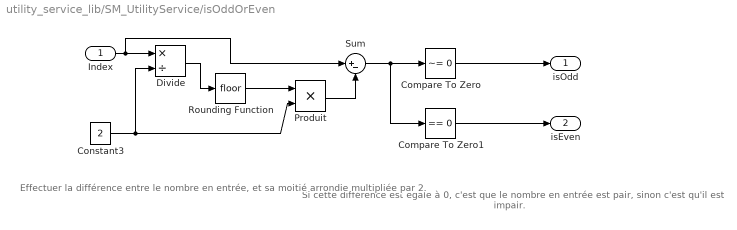
== system utility_service_lib/SM_UtilityService/isOddOrEven ==
  note: Si cette différence est égale à 0, c'est que le
      | nombre en entrée est pair, sinon c'est qu'il est impair.
  note: Effectuer la différence entre le nombre en entrée,
      | et sa moitié arrondie multipliée par 2.
  Index : Inport
  Compare To Zero : simulink/Logic and Bit Operations/Compare To Zero  relop=~=  OutDataTypeStr=boolean  ZeroCross=off
  Compare To Zero1 : simulink/Logic and Bit Operations/Compare To Zero  relop===  OutDataTypeStr=boolean  ZeroCross=off
  Constant3 : Constant  Value=2
  Divide : Product  Inputs=*/  OutDataTypeStr=double
  Produit : Product  Inputs=**  OutDataTypeStr=double
  Rounding Function : Rounding
  Sum : Sum  Inputs=|+-
  isOdd : Outport
  isEven : Outport  Port=2
  wires:
  Compare To Zero1/1 -> isEven/1
  Compare To Zero/1 -> isOdd/1
  Sum/1 -> Compare To Zero1/1, Compare To Zero/1
  Produit/1 -> Sum/2
  Rounding Function/1 -> Produit/1
  Index/1 -> Sum/1, Divide/1
  Divide/1 -> Rounding Function/1
  Constant3/1 -> Produit/2, Divide/2

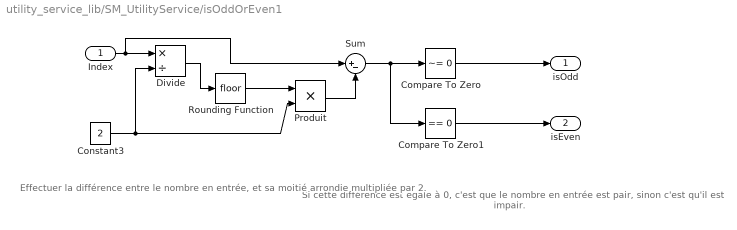
== system utility_service_lib/SM_UtilityService/isOddOrEven1 ==
  note: Si cette différence est égale à 0, c'est que le
      | nombre en entrée est pair, sinon c'est qu'il est impair.
  note: Effectuer la différence entre le nombre en entrée,
      | et sa moitié arrondie multipliée par 2.
  Index : Inport
  Compare To Zero : simulink/Logic and Bit Operations/Compare To Zero  relop=~=  OutDataTypeStr=boolean  ZeroCross=off
  Compare To Zero1 : simulink/Logic and Bit Operations/Compare To Zero  relop===  OutDataTypeStr=boolean  ZeroCross=off
  Constant3 : Constant  Value=2
  Divide : Product  Inputs=*/  OutDataTypeStr=double
  Produit : Product  Inputs=**  OutDataTypeStr=double
  Rounding Function : Rounding
  Sum : Sum  Inputs=|+-
  isOdd : Outport
  isEven : Outport  Port=2
  wires:
  Compare To Zero1/1 -> isEven/1
  Compare To Zero/1 -> isOdd/1
  Sum/1 -> Compare To Zero1/1, Compare To Zero/1
  Produit/1 -> Sum/2
  Rounding Function/1 -> Produit/1
  Index/1 -> Sum/1, Divide/1
  Divide/1 -> Rounding Function/1
  Constant3/1 -> Produit/2, Divide/2

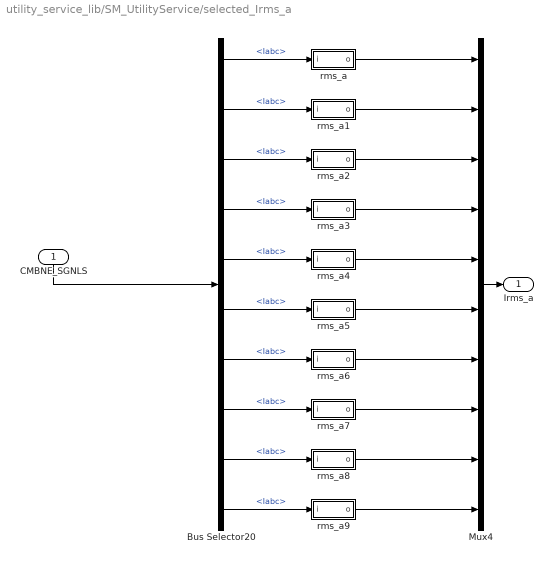
== system utility_service_lib/SM_UtilityService/selected_Irms_a ==
  CMBNE_SGNLS : Inport
  Bus Selector20 : BusSelector  OutputSignals=F3_MS_IN.CB_DATA.F3_PCC.Iabc,F3_MS_IN.CB_DATA.F3_CB_3.Iabc,F2_MS_IN.CB_DATA.F2_PCC.Iabc,F2_MS_IN.CB_DATA.F2_CB_1.Iabc,F2_MS_IN.CB_DATA.F2_CB_3.Iabc,F1_MS_IN.CB_DATA.F1_PCC.Iabc,F1_MS_IN.DIESEL_DATA.DIESEL_GCB.cb_ms.Iabc,F1_MS_IN.CB_DATA.F1_CB_2.Iabc,F1_MS_IN.CB_DATA.F1_CB_3.Iabc,F1_MS_IN.CB_DATA.F1_CB_6.Iabc
  Mux4 : Mux  Inputs=10
  rms_a : Subsystem
  rms_a1 : Subsystem
  rms_a2 : Subsystem
  rms_a3 : Subsystem
  rms_a4 : Subsystem
  rms_a5 : Subsystem
  rms_a6 : Subsystem
  rms_a7 : Subsystem
  rms_a8 : Subsystem
  rms_a9 : Subsystem
  Irms_a : Outport
  wires:
  Bus Selector20/4 -> rms_a3/1(i)  "<Iabc>"
  Bus Selector20/8 -> rms_a7/1(i)  "<Iabc>"
  rms_a2/1(o) -> Mux4/3
  CMBNE_SGNLS/1 -> Bus Selector20/1
  Bus Selector20/3 -> rms_a2/1(i)  "<Iabc>"
  rms_a4/1(o) -> Mux4/5
  rms_a7/1(o) -> Mux4/8
  rms_a8/1(o) -> Mux4/9
  rms_a3/1(o) -> Mux4/4
  rms_a9/1(o) -> Mux4/10
  Mux4/1 -> Irms_a/1
  rms_a6/1(o) -> Mux4/7
  Bus Selector20/5 -> rms_a4/1(i)  "<Iabc>"
  rms_a1/1(o) -> Mux4/2
  rms_a5/1(o) -> Mux4/6
  Bus Selector20/10 -> rms_a9/1(i)  "<Iabc>"
  rms_a/1(o) -> Mux4/1
  Bus Selector20/7 -> rms_a6/1(i)  "<Iabc>"
  Bus Selector20/9 -> rms_a8/1(i)  "<Iabc>"
  Bus Selector20/2 -> rms_a1/1(i)  "<Iabc>"
  Bus Selector20/1 -> rms_a/1(i)  "<Iabc>"
  Bus Selector20/6 -> rms_a5/1(i)  "<Iabc>"

== system utility_service_lib/SM_UtilityService/Number of seconds of recording/Increment ==
  Trigger : TriggerPort
  Increment : Constant
  Memory : Memory  InheritSampleTime=on
  Sum : Sum  Inputs=|++
  Out1 : Outport
  wires:
  Sum/1 -> Out1/1, Memory/1
  Memory/1 -> Sum/1
  Increment/1 -> Sum/2

== system utility_service_lib/SM_UtilityService/Number of seconds of recording1/Increment ==
  Trigger : TriggerPort
  Increment : Constant
  Memory : Memory  InheritSampleTime=on
  Sum : Sum  Inputs=|++
  Out1 : Outport
  wires:
  Sum/1 -> Out1/1, Memory/1
  Memory/1 -> Sum/1
  Increment/1 -> Sum/2

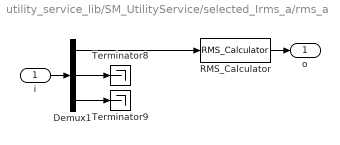
== system utility_service_lib/SM_UtilityService/selected_Irms_a/rms_a ==
  i : Inport
  Demux1 : Demux  Outputs=3
  RMS_Calculator : RMS_lib/RMS_Calculator
  Terminator8 : Terminator
  Terminator9 : Terminator
  o : Outport
  wires:
  Demux1/3 -> Terminator9/1
  Demux1/2 -> Terminator8/1
  Demux1/1 -> RMS_Calculator/1
  RMS_Calculator/1 -> o/1
  i/1 -> Demux1/1

== system utility_service_lib/SM_UtilityService/selected_Irms_a/rms_a1 ==
  i : Inport
  Demux1 : Demux  Outputs=3
  RMS_Calculator : RMS_lib/RMS_Calculator
  Terminator8 : Terminator
  Terminator9 : Terminator
  o : Outport
  wires:
  Demux1/3 -> Terminator9/1
  Demux1/2 -> Terminator8/1
  Demux1/1 -> RMS_Calculator/1
  RMS_Calculator/1 -> o/1
  i/1 -> Demux1/1

== system utility_service_lib/SM_UtilityService/selected_Irms_a/rms_a2 ==
  i : Inport
  Demux1 : Demux  Outputs=3
  RMS_Calculator : RMS_lib/RMS_Calculator
  Terminator8 : Terminator
  Terminator9 : Terminator
  o : Outport
  wires:
  Demux1/3 -> Terminator9/1
  Demux1/2 -> Terminator8/1
  Demux1/1 -> RMS_Calculator/1
  RMS_Calculator/1 -> o/1
  i/1 -> Demux1/1

== system utility_service_lib/SM_UtilityService/selected_Irms_a/rms_a3 ==
  i : Inport
  Demux1 : Demux  Outputs=3
  RMS_Calculator : RMS_lib/RMS_Calculator
  Terminator8 : Terminator
  Terminator9 : Terminator
  o : Outport
  wires:
  Demux1/3 -> Terminator9/1
  Demux1/2 -> Terminator8/1
  Demux1/1 -> RMS_Calculator/1
  RMS_Calculator/1 -> o/1
  i/1 -> Demux1/1

== system utility_service_lib/SM_UtilityService/selected_Irms_a/rms_a4 ==
  i : Inport
  Demux1 : Demux  Outputs=3
  RMS_Calculator : RMS_lib/RMS_Calculator
  Terminator8 : Terminator
  Terminator9 : Terminator
  o : Outport
  wires:
  Demux1/3 -> Terminator9/1
  Demux1/2 -> Terminator8/1
  Demux1/1 -> RMS_Calculator/1
  RMS_Calculator/1 -> o/1
  i/1 -> Demux1/1

== system utility_service_lib/SM_UtilityService/selected_Irms_a/rms_a5 ==
  i : Inport
  Demux1 : Demux  Outputs=3
  RMS_Calculator : RMS_lib/RMS_Calculator
  Terminator8 : Terminator
  Terminator9 : Terminator
  o : Outport
  wires:
  Demux1/3 -> Terminator9/1
  Demux1/2 -> Terminator8/1
  Demux1/1 -> RMS_Calculator/1
  RMS_Calculator/1 -> o/1
  i/1 -> Demux1/1

== system utility_service_lib/SM_UtilityService/selected_Irms_a/rms_a6 ==
  i : Inport
  Demux1 : Demux  Outputs=3
  RMS_Calculator : RMS_lib/RMS_Calculator
  Terminator8 : Terminator
  Terminator9 : Terminator
  o : Outport
  wires:
  Demux1/3 -> Terminator9/1
  Demux1/2 -> Terminator8/1
  Demux1/1 -> RMS_Calculator/1
  RMS_Calculator/1 -> o/1
  i/1 -> Demux1/1

== system utility_service_lib/SM_UtilityService/selected_Irms_a/rms_a7 ==
  i : Inport
  Demux1 : Demux  Outputs=3
  RMS_Calculator : RMS_lib/RMS_Calculator
  Terminator8 : Terminator
  Terminator9 : Terminator
  o : Outport
  wires:
  Demux1/3 -> Terminator9/1
  Demux1/2 -> Terminator8/1
  Demux1/1 -> RMS_Calculator/1
  RMS_Calculator/1 -> o/1
  i/1 -> Demux1/1

== system utility_service_lib/SM_UtilityService/selected_Irms_a/rms_a8 ==
  i : Inport
  Demux1 : Demux  Outputs=3
  RMS_Calculator : RMS_lib/RMS_Calculator
  Terminator8 : Terminator
  Terminator9 : Terminator
  o : Outport
  wires:
  Demux1/3 -> Terminator9/1
  Demux1/2 -> Terminator8/1
  Demux1/1 -> RMS_Calculator/1
  RMS_Calculator/1 -> o/1
  i/1 -> Demux1/1

== system utility_service_lib/SM_UtilityService/selected_Irms_a/rms_a9 ==
  i : Inport
  Demux1 : Demux  Outputs=3
  RMS_Calculator : RMS_lib/RMS_Calculator
  Terminator8 : Terminator
  Terminator9 : Terminator
  o : Outport
  wires:
  Demux1/3 -> Terminator9/1
  Demux1/2 -> Terminator8/1
  Demux1/1 -> RMS_Calculator/1
  RMS_Calculator/1 -> o/1
  i/1 -> Demux1/1
